simulink model "ssc_lithium_cell_2RC"  (Simulink 7.9)
settings: Solver=ode15s  StartTime=0.0  StopTime=40000  RelTol=1e-3
PreLoadFcn:
  | ssc_lithium_cell_2RC_ini
values from neighbouring files (symbols this model uses):
  C1_LUT = [ ... (first row only)    [ssc_lithium_cell_1RC_ini.m]
  Capacity_LUT = [ ... (first row only)    [ssc_lithium_cell_1RC_ini.m]
  cell_Cp_heat = cell_rho_Cp * cell_volume    (= 810.5328)    [ssc_lithium_cell_1RC_ini.m]
  cell_mass = 1    [ssc_lithium_cell_1RC_ini.m]
  Em_LUT = [ ... (first row only)    [ssc_lithium_cell_1RC_ini.m]
  Qe_init = 15.6845    [ssc_lithium_cell_1RC_ini.m]
  R0_LUT = [ ... (first row only)    [ssc_lithium_cell_1RC_ini.m]
  R1_LUT = [ ... (first row only)    [ssc_lithium_cell_1RC_ini.m]
  SOC_LUT = [0 0.1 0.25 0.5 0.75 0.9 1]'    [ssc_lithium_cell_1RC_ini.m]
  T_init = 20 + 273.15    (= 293.15)    [ssc_lithium_cell_1RC_ini.m]
  Temperature_LUT = [5 20 40] + 273.15    [ssc_lithium_cell_1RC_ini.m]
undefined symbols (not defined in the file or in its folder): C2_LUT, R2_LUT, sigbuilder_block
libraries: fl_lib x13, nesl_utility x6, LiBatteryElements_lib x6
Description:
  | Lithium Battery Cell - 2 RC Branch Equivalent Circuit
  | 
  | This demo implements a model of a lithium cell using the Simscape language to implement the elements of an equivalent circuit model with two RC branches. For the defining equations and their validation, see T. Huria, M. Ceraolo, J. Gazzarri, R. Jackey. "High Fidelity Electrical Model with Thermal Dependence for Characterization and Simulation of High Power Lithium Battery Cells," IEEE International Electric Vehicle Conference, March 2012.
  | 
  | A simple thermal model is used to model battery temperature. It is assumed that cooling is primarily via convection, and that heating is primarily from internal resistance. A battery pack can be modeled by connecting multiple copies of the battery cell block in series.
  | 
  | Copyright 2012 The MathWorks, Inc.
settings Model: Creator=MathWorks  LastModifiedBy=rjackey
settings DataIOCC: SaveOutput=off  SaveTime=off
settings DebuggingCC: SolverPrmCheckMsg=none  FcnCallInpInsideContextMsg=Use local settings  StrictBusMsg=Warning
settings GRTTargetCC: CombineOutputUpdateFcns=off  GRTInterface=on

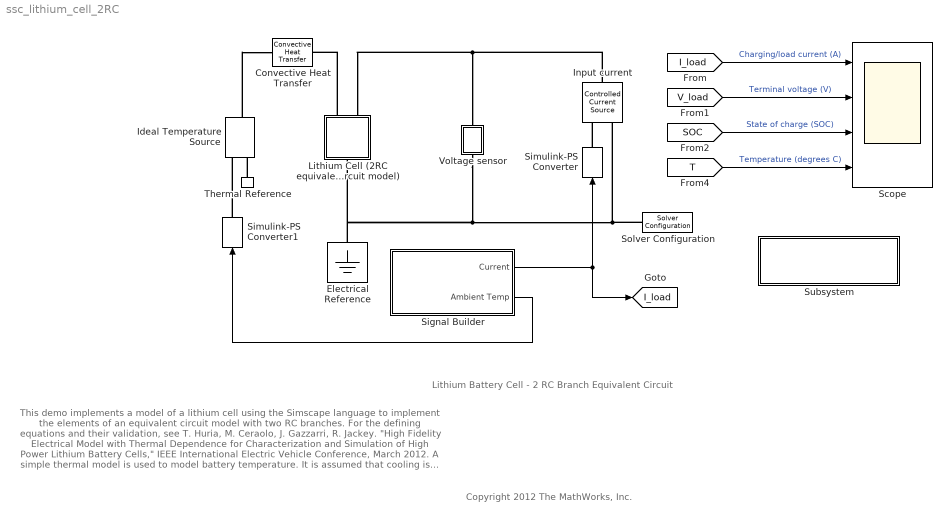
== system ssc_lithium_cell_2RC ==
  note: Lithium Battery Cell - 2 RC Branch Equivalent Circuit
  note: This demo implements a model of a lithium cell using the Simscape language to implement the elements of an equivalent circuit model with two
      | RC branches. For the defining equations and their validation, see T. Huria, M. Ceraolo, J. Gazzarri, R. Jackey. "High Fidelity Electrical Model with
      | Thermal Dependence for Characterization and Simulation of High Power Lithium Battery Cells," IEEE International Electric Vehicle Conference,
      | March 2012. A simple thermal model is used to model battery temperature. It is assumed that cooling is primarily via convection, and that heating
      | is primarily from internal resistance. A battery pack can be modeled by connecting multiple copies of the battery cell block in series.
  note: Copyright 2012 The MathWorks, Inc.
  Convective Heat Transfer : fl_lib/Thermal/Thermal Elements/Convective Heat Transfer  area=cell_area m^2  heat_tr_coeff=h_conv W/(m^2 * K)  Q_Log=off  T_Log=off  LocalVarNames=|heat_flow|temperature_diff  LocalVarDescs=|Heat flow (J/s)|Temperature difference (K)  LocalVarLogging=[0 0]
  Electrical Reference : fl_lib/Electrical/Electrical Elements/Electrical Reference  i_Log=off  LocalVarNames=|i  LocalVarDescs=|i  LocalVarLogging=[]
  Ideal Temperature Source : fl_lib/Thermal/Thermal Sources/Ideal Temperature Source  Q_Log=off  T_Log=off  LocalVarNames=|heat_flow|T_differential  LocalVarDescs=|Heat flow rate through the source (J/s)|Temperature differential across the source (K)  LocalVarLogging=[0 0]
  Input current : fl_lib/Electrical/Electrical Sources/Controlled Current Source  i_Log=off  v_Log=off  LocalVarNames=|current|voltage|power  LocalVarDescs=|Current (A)|Voltage (V)|Power (W)  LocalVarLogging=[0 0 0]
  Lithium Cell (2RC equivalent circuit model) : Subsystem  mask{Qe_init=Qe_init, T_init=T_init, Capacity_LUT=Capacity_LUT, Em_LUT=Em_LUT, R0_LUT=R0_LUT, R1_LUT=R1_LUT, C1_LUT=C1_LUT, R2_LUT=R2_LUT, C2_LUT=C2_LUT, cell_mass=cell_mass, cell_Cp_heat=cell_Cp_heat, SOC_LUT=SOC_LUT, Temperature_LUT=Temperature_LUT}
      mask prompts: Qe_init "Initial Charge Deficit (A*hr)"; T_init "Initial Cell Temperature (K)"; Capacity_LUT "Capacity (A*hr, 1xN table)"; Em_LUT "Em Open-Circuit Voltage (MxN table)"; R0_LUT "R0: Terminal Resistance (Ohms, MxN table)"; R1_LUT "R1 Resistance (Ohms, MxN table)"; C1_LUT "C1 Capacitance (Farads, MxN table)"; R2_LUT "R2 Resistance (Ohms, MxN table)"; C2_LUT "C2 Capacitance (Farads, MxN table)"; cell_mass "Cell Mass (kg)"; cell_Cp_heat "Cell Specific Heat (J/kg/K)"; SOC_LUT "SOC Table Breakpoints (Mx1 array)"; Temperature_LUT "Temperature Table Breakpoints(K, 1xN array)"
      mask TabNameString: Initial Conditions,Initial Conditions,Electrical,Electrical,Electrical,Electrical,Electrical,Electrical,Electrical,Thermal,Thermal,Table Breakpoints,Table Breakpoints
      mask Display:
      | image(imread('battery.jpg'))
      | color('red')
      | port_label('LConn',1,'H')
      | port_label('LConn',2,'+')
      | port_label('RConn',1,'-')
  Scope : Scope  NumInputPorts=4
      settings: TimeRange=40000  YMin=-4.5~2.6~0~20  YMax=3.5~3.7~1~30
  Signal Builder : Subsystem  Tag=STV Subsys  LoadFcn=sigbuilder_block('load');  StartFcn=sigbuilder_block('start');  StopFcn=sigbuilder_block('stop');  ClipboardFcn=sigbuilder_block('clipboard');  mask(Sigbuilder block){}
      mask help: Simulink:masks:SigbuilderBlock_MD
      mask init:
      | if ~strcmp(get_param(bdroot(gcbh),'SimulationStatus'),'stopped') tuvar = sigbuilder_block('maskInit'); end
      settings: CopyFcn=sigbuilder_block('copy');  DeleteFcn=sigbuilder_block('delete');  ModelCloseFcn=sigbuilder_block('modelClose');  PreSaveFcn=sigbuilder_block('preSave');  PauseFcn=sigbuilder_block('pause');  ContinueFcn=sigbuilder_block('continue');  NameChangeFcn=sigbuilder_block('namechange');  OpenFcn=sigbuilder_block('open',[62.25 82.5 550.5 303 ]);  CloseFcn=sigbuilder_block('close');
      mask Display: plot(0, 0, 100, 100,[2, 2, 32, 32, 2], [68, 8, 8, 68, 68],[32, 2], [38, 38], [32, 19, 2],[53, 60, 44], [32, 17, 17, 2],[16, 16, 31, 31]);txt = getActiveGroup(gcbh);text(2, 100, txt,'verticalAlignment', 'top');
  Simulink-PS Converter : nesl_utility/Simulink-PS Converter  PhysicalDomain=network_engine_domain  LeftPortType=input  RightPortType=output  SubClassName=ps_input  Unit=A  AffineConversion=on  InputFilterTimeConstant=.001  UdotUserProvided=1  SimscapeFilterOrder=1  InputFiltering=off
  Simulink-PS Converter1 : nesl_utility/Simulink-PS Converter  PhysicalDomain=network_engine_domain  LeftPortType=input  RightPortType=output  SubClassName=ps_input  Unit=C  AffineConversion=on  InputFilterTimeConstant=.001  UdotUserProvided=1  SimscapeFilterOrder=1  InputFiltering=off
  Solver Configuration : nesl_utility/Solver Configuration  PhysicalDomain=network_engine_domain  LeftPortType=input  RightPortType=generic  SubClassName=solver  UseCustomDae=off  DoDC=off  ResidualTolerance=1e-9  UseLocalSolver=off  LocalSolverChoice=NE_BACKWARD_EULER_ADVANCER  LocalSolverSampleTime=.001  DoFixedCost=off  MaxNonlinIter=3  MaxModeIter=2  LinearAlgebra=Sparse  Accelerate=off  Profile=off  UseLocalSampling=off  DelaysMemoryBudget=1024
  Subsystem : Subsystem
      settings: OpenFcn=open('LiBatteryElements_lib.mdl')
      mask Display: disp('Open the custom\n library used by the\n Lithium Cell block')
  Thermal Reference : fl_lib/Thermal/Thermal Elements/Thermal Reference  Q_Log=off  LocalVarNames=|Q  LocalVarDescs=|Q  LocalVarLogging=[]
  Voltage sensor : Subsystem
  tag scope: I_load=global
  wires:
  [SOC] -> Scope/3  "State of charge (SOC)"
  [T] -> Scope/4  "Temperature (degrees C)"
  [I_load] -> Scope/1  "Charging/load current (A)"
  [V_load] -> Scope/2  "Terminal voltage (V)"
  Signal Builder/2(Ambient Temp) -> Simulink-PS Converter1/1
  Signal Builder/1(Current) -> Simulink-PS Converter/1, [I_load]
  connections:
  Electrical Reference/LConn1 -- Lithium Cell (2RC equivalent circuit model)/RConn1 -- Solver Configuration/RConn1 -- Input current/RConn2 -- Voltage sensor/RConn1
  Input current/LConn1 -- Lithium Cell (2RC equivalent circuit model)/LConn2 -- Voltage sensor/LConn1
  Thermal Reference/LConn1 -- Ideal Temperature Source/RConn2
  Ideal Temperature Source/LConn1 -- Convective Heat Transfer/LConn1
  Lithium Cell (2RC equivalent circuit model)/LConn1 -- Convective Heat Transfer/RConn1
  Simulink-PS Converter/RConn1 -- Input current/RConn1
  Simulink-PS Converter1/RConn1 -- Ideal Temperature Source/RConn1

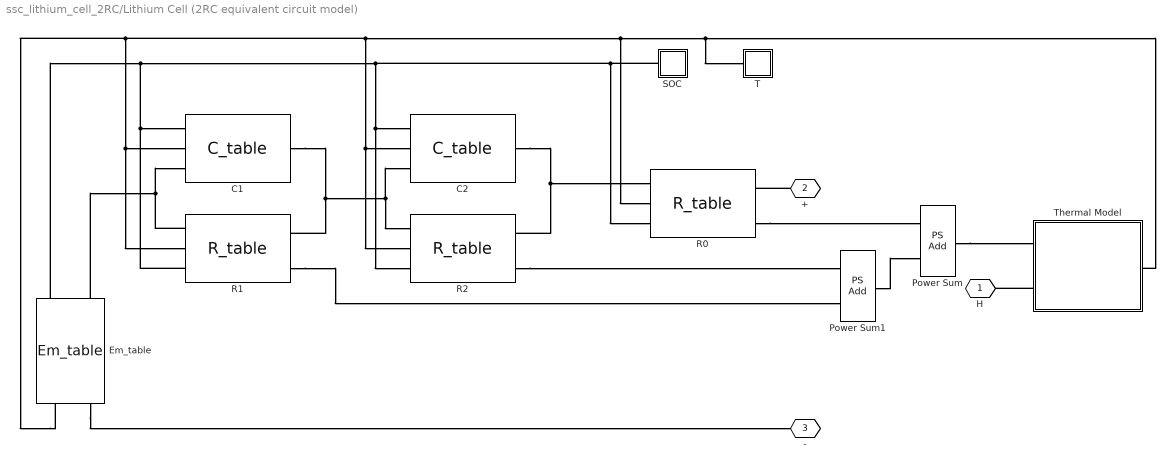
== system ssc_lithium_cell_2RC/Lithium Cell (2RC equivalent circuit model) ==
  " SOC " : Subsystem
  C1 : LiBatteryElements_lib/C_table  C_Table=C1_LUT F  SOC_Table=SOC_LUT  Temp_Table=Temperature_LUT K  v0=0 V  i_Log=off  v_Log=off  LocalVarNames=|i|v  LocalVarDescs=|i|v  LocalVarLogging=[0 0]
  C2 : LiBatteryElements_lib/C_table  C_Table=C2_LUT F  SOC_Table=SOC_LUT  Temp_Table=Temperature_LUT K  v0=0 V  i_Log=off  v_Log=off  LocalVarNames=|i|v  LocalVarDescs=|i|v  LocalVarLogging=[0 0]
  Em_table : LiBatteryElements_lib/Em_table  C_Table=Capacity_LUT hr*A  Em_Table=Em_LUT V  SOC_Table=SOC_LUT  Temp_Table=Temperature_LUT K  Qinit=Qe_init hr*A  i_Log=off  v_Log=off  Qe_Log=off  LocalVarNames=|i|v|Qe  LocalVarDescs=|i|v|Charge deficit  LocalVarLogging=[0 0 0]
  Power Sum : fl_lib/Physical Signals/Functions/PS Add  LocalVarLogging=[]
  Power Sum1 : fl_lib/Physical Signals/Functions/PS Add  LocalVarLogging=[]
  R0 : LiBatteryElements_lib/R_table  R_Table=R0_LUT Ohm  SOC_Table=SOC_LUT  Temp_Table=Temperature_LUT K  i_Log=off  v_Log=off  LocalVarNames=|i|v  LocalVarDescs=|i|v  LocalVarLogging=[0 0]
  R1 : LiBatteryElements_lib/R_table  R_Table=R1_LUT Ohm  SOC_Table=SOC_LUT  Temp_Table=Temperature_LUT K  i_Log=off  v_Log=off  LocalVarNames=|i|v  LocalVarDescs=|i|v  LocalVarLogging=[0 0]
  R2 : LiBatteryElements_lib/R_table  R_Table=R2_LUT Ohm  SOC_Table=SOC_LUT  Temp_Table=Temperature_LUT K  i_Log=off  v_Log=off  LocalVarNames=|i|v  LocalVarDescs=|i|v  LocalVarLogging=[0 0]
  T : Subsystem
  Thermal Model : Subsystem
  H : PMIOPort  Tag=PMCPort  Port=1  Side=Left
  + : PMIOPort  Tag=PMCPort  Port=2  Side=Left
  - : PMIOPort  Tag=PMCPort  Port=3  Side=Right
  connections:
  Thermal Model/LConn2 -- H/RConn1
  Em_table/RConn1 -- -/RConn1
  +/RConn1 -- R0/RConn1
  Em_table/LConn1 -- C1/LConn1 -- R1/LConn1
  C2/LConn2 -- R2/LConn2 -- Em_table/RConn2 -- C1/LConn2 -- R1/LConn2 -- Thermal Model/RConn1 -- T/LConn1 -- R0/LConn2
  Power Sum/RConn1 -- Thermal Model/LConn1
  C1/RConn1 -- R1/RConn1 -- C2/LConn1 -- R2/LConn1
  R0/RConn2 -- Power Sum/LConn1
  Power Sum1/RConn1 -- Power Sum/LConn2
  C2/RConn1 -- R2/RConn1 -- R0/LConn1
  R2/RConn2 -- Power Sum1/LConn1
  R1/LConn3 -- C1/LConn3 -- Em_table/LConn3 -- " SOC "/LConn1 -- R0/LConn3 -- C2/LConn3 -- R2/LConn3
  R1/RConn2 -- Power Sum1/LConn2

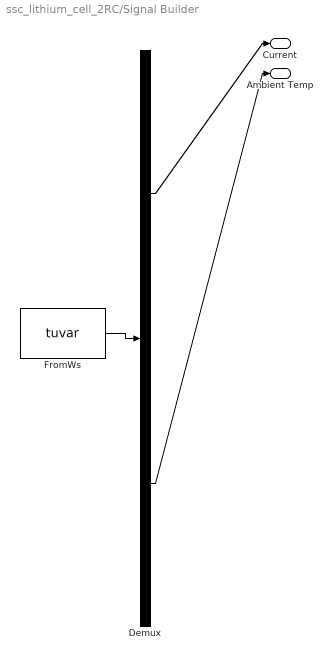
== system ssc_lithium_cell_2RC/Signal Builder ==
  Demux : Demux  Tag=STV Demux  Outputs=2
  FromWs : FromWorkspace  Tag=STV FromWs  VariableName=tuvar  SampleTime=0  SigBuilderData=DataTag0  VnvData=DataTag1
      SigBuilderData=|
      | common.afterFinalStr = 'Extrapolate'
      | common.sampleTime = 0
      | dataSet(1).timeRange = [0 40000]
      | dataSet(1).name = 'Pulse'
      | dataSet(2).timeRange = [0 40000]
      | dataSet(2).name = 'Constant'
      | sbobj.Name = 'Signal Builder'
      | sbobj.Groups(1).Name = 'Pulse'
      | sbobj.Groups(1).Signals(1).Name = 'Current'
      | sbobj.Groups(1).Signals(1).XData = [0 300 300 1215 1215 3600 3600 3960 3960 7200 7200 7560 7560 10800 10800 11160 11160 14400 14400 14760 14760 18000 18000 18360 18360 21600 21600 21960 21960 25200 25200 25560 25560 28800 28800 29160 29160 32400 32400 32760 32760 36000 36000 36360 36360 40000]
      | sbobj.Groups(1).Signals(1).YData = [0 0 3.15 3.15 0 0 -4.18 -4.18 0 0 -4.18 -4.18 0 0 -4.18 -4.18 0 0 -4.18 -4.18 0 0 -4.18 -4.18 0 0 -4.18 -4.18 0 0 -4.18 -4.18 0 0 -4.18 -4.18 0 0 -4.18 -4.18 0 0 -4.18 -4.18 0 0]
      | sbobj.Groups(1).Signals(2).Name = 'Ambient Temp'
      | sbobj.Groups(1).Signals(2).XData = [0 300 300 1215 1215 3600 3600 3960 3960 7200 7200 7560 7560 10800 10800 11160 11160 14400 14400 14760 14760 18000 18000 18360 18360 21600 21600 21960 21960 25200 25200 25560 25560 28800 28800 29160 29160 32400 32400 32760 32760 36000 36000 36360 36360 40000]
      | sbobj.Groups(1).Signals(2).YData = [20 20 20 20 20 20 20 20 20 20 20 20 20 20 20 20 20 20 20 20 20 20 20 20 20 20 20 20 20 20 20 20 20 20 20 20 20 20 20 20 20 20 20 20 20 20]
      | sbobj.Groups(1).TimeRange = [0 40000]
      | sbobj.Groups(2).Name = 'Constant'
      | sbobj.Groups(2).Signals(1).Name = 'Current'
      | sbobj.Groups(2).Signals(1).XData = [0 360 360 12500 12500 15800 15800 26500 34500 40000]
      | sbobj.Groups(2).Signals(1).YData = [0 0 -1 -1 0 0 1 1 0 0]
      | sbobj.Groups(2).Signals(2).Name = 'Ambient Temp'
      | sbobj.Groups(2).Signals(2).XData = [0 360 360 12500 12500 15800 15800 26500 34500 40000]
      | sbobj.Groups(2).Signals(2).YData = [20 20.09 20.09 23.125 23.125 23.95 23.95 26.625 28.625 30]
      | sbobj.Groups(2).TimeRange = [0 40000]
  Current : Outport
  Ambient Temp : Outport  Tag=STV Outport  Port=2
  wires:
  FromWs/1 -> Demux/1
  Demux/1 -> Current/1
  Demux/2 -> Ambient Temp/1

== system ssc_lithium_cell_2RC/Subsystem ==

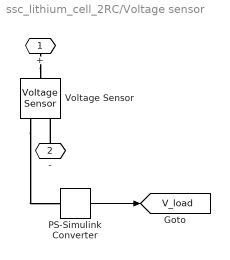
== system ssc_lithium_cell_2RC/Voltage sensor ==
  PS-Simulink Converter : nesl_utility/PS-Simulink Converter  PhysicalDomain=network_engine_domain  LeftPortType=input  RightPortType=output  SubClassName=ps_output  Unit=V  AffineConversion=off
  Voltage Sensor : fl_lib/Electrical/Electrical Sensors/Voltage Sensor  i1_Log=off  v1_Log=off  LocalVarNames=|i1|v1  LocalVarDescs=|i1|v1  LocalVarLogging=[]
  + : PMIOPort  Port=1  Side=Left
  - : PMIOPort  Port=2  Side=Right
  tag scope: V_load=global
  wires:
  PS-Simulink Converter/1 -> [V_load]
  connections:
  Voltage Sensor/RConn1 -- PS-Simulink Converter/LConn1
  +/RConn1 -- Voltage Sensor/LConn1
  -/RConn1 -- Voltage Sensor/RConn2

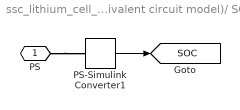
== system ssc_lithium_cell_2RC/Lithium Cell (2RC equivalent circuit model)/ SOC  ==
  PS-Simulink Converter1 : nesl_utility/PS-Simulink Converter  PhysicalDomain=network_engine_domain  LeftPortType=input  RightPortType=output  SubClassName=ps_output  Unit=1  AffineConversion=off
  PS : PMIOPort  Port=1  Side=Left
  tag scope: SOC=global
  wires:
  PS-Simulink Converter1/1 -> [SOC]
  connections:
  PS/RConn1 -- PS-Simulink Converter1/LConn1

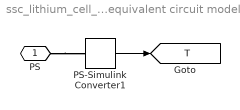
== system ssc_lithium_cell_2RC/Lithium Cell (2RC equivalent circuit model)/T ==
  PS-Simulink Converter1 : nesl_utility/PS-Simulink Converter  PhysicalDomain=network_engine_domain  LeftPortType=input  RightPortType=output  SubClassName=ps_output  Unit=C  AffineConversion=on
  PS : PMIOPort  Port=1  Side=Left
  tag scope: T=global
  wires:
  PS-Simulink Converter1/1 -> [T]
  connections:
  PS/RConn1 -- PS-Simulink Converter1/LConn1

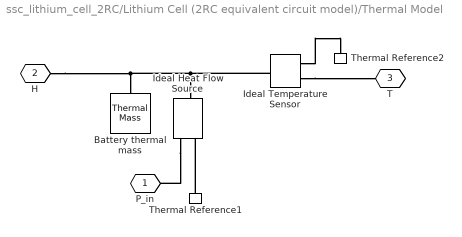
== system ssc_lithium_cell_2RC/Lithium Cell (2RC equivalent circuit model)/Thermal Model ==
  Battery thermal mass : fl_lib/Thermal/Thermal Elements/Thermal Mass  mass=cell_mass kg  sp_heat=cell_Cp_heat J/kg/K  init_temp=T_init K  Q_Log=off  LocalVarNames=|heat_flow|temperature  LocalVarDescs=|Heat flow (J/s)|Mass temperature (K)  LocalVarLogging=[0 0]
  Ideal Temperature Sensor : fl_lib/Thermal/Thermal Sensors/Ideal Temperature Sensor  Qs_Log=off  Ts_Log=off  LocalVarNames=|Qs|Ts  LocalVarDescs=|Qs|Ts  LocalVarLogging=[]
  Ideal Heat Flow Source : fl_lib/Thermal/Thermal Sources/Ideal Heat Flow Source  Q_Log=off  T_Log=off  LocalVarNames=|heat_flow|T_differential  LocalVarDescs=|Heat flow through the source (J/s)|Temperature differential across the source (K)  LocalVarLogging=[0 0]
  Thermal Reference1 : fl_lib/Thermal/Thermal Elements/Thermal Reference  Q_Log=off  LocalVarNames=|Q  LocalVarDescs=|Q  LocalVarLogging=[]
  Thermal Reference2 : fl_lib/Thermal/Thermal Elements/Thermal Reference  Q_Log=off  LocalVarNames=|Q  LocalVarDescs=|Q  LocalVarLogging=[]
  P_in : PMIOPort  Tag=PMCPort  Port=1  Side=Left
  H : PMIOPort  Tag=PMCPort  Port=2  Side=Left
  T : PMIOPort  Tag=PMCPort  Port=3  Side=Right
  connections:
  Ideal Temperature Sensor/RConn1 -- Thermal Reference2/LConn1
  Ideal Temperature Sensor/RConn2 -- T/RConn1
  Thermal Reference1/LConn1 -- Ideal Heat Flow Source/RConn2
  Ideal Temperature Sensor/LConn1 -- H/RConn1 -- Battery thermal mass/LConn1 -- Ideal Heat Flow Source/LConn1
  Ideal Heat Flow Source/RConn1 -- P_in/RConn1
